simulink model "TST_Rail_CtlLoop"  (R2016b)
settings: Solver=FixedStepDiscrete  StartTime=0.0  StopTime=simTime  FixedStep=sampleTime  RelTol=1e-3
values from neighbouring files (symbols this model uses):
  testCase = 1    [initTST_Rail_CtlLoop_001.m]
libraries: simulink x6, UnitTest_Lib x4
settings Model: Creator=zhengjinyan  LastModifiedBy=zhengjinyan
settings DebuggingCC: SignalRangeChecking=error

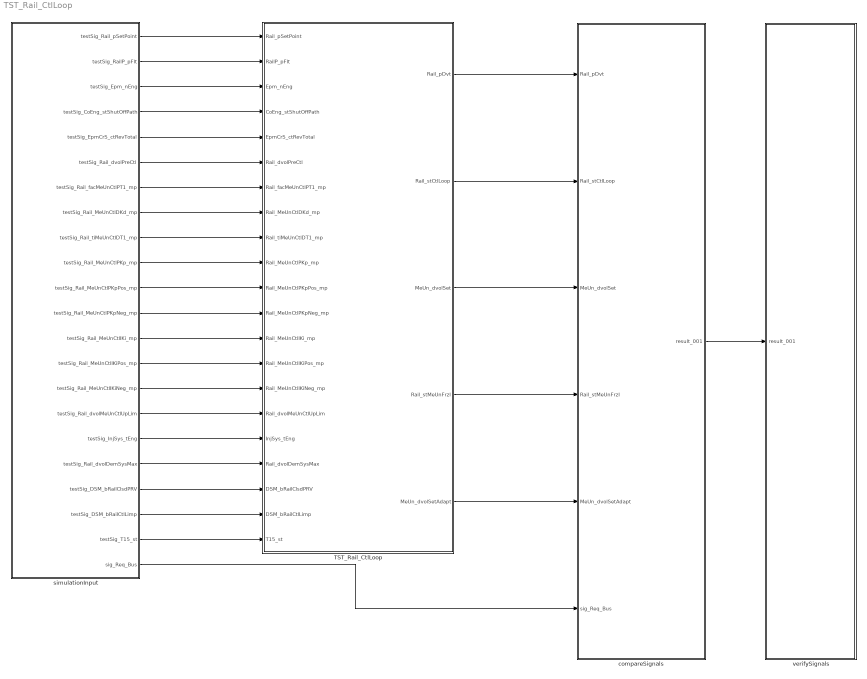
== system TST_Rail_CtlLoop ==
  TST_Rail_CtlLoop : Subsystem
  compareSignals : Subsystem
  simulationInput : Subsystem
  verifySignals : Subsystem
  wires:
  simulationInput/1(testSig_Rail_pSetPoint) -> TST_Rail_CtlLoop/1(Rail_pSetPoint)
  simulationInput/2(testSig_RailP_pFlt) -> TST_Rail_CtlLoop/2(RailP_pFlt)
  simulationInput/3(testSig_Epm_nEng) -> TST_Rail_CtlLoop/3(Epm_nEng)
  simulationInput/4(testSig_CoEng_stShutOffPath) -> TST_Rail_CtlLoop/4(CoEng_stShutOffPath)
  simulationInput/5(testSig_EpmCrS_ctRevTotal) -> TST_Rail_CtlLoop/5(EpmCrS_ctRevTotal)
  simulationInput/6(testSig_Rail_dvolPreCtl) -> TST_Rail_CtlLoop/6(Rail_dvolPreCtl)
  simulationInput/7(testSig_Rail_facMeUnCtlPT1_mp) -> TST_Rail_CtlLoop/7(Rail_facMeUnCtlPT1_mp)
  simulationInput/8(testSig_Rail_MeUnCtlDKd_mp) -> TST_Rail_CtlLoop/8(Rail_MeUnCtlDKd_mp)
  simulationInput/9(testSig_Rail_tiMeUnCtlDT1_mp) -> TST_Rail_CtlLoop/9(Rail_tiMeUnCtlDT1_mp)
  simulationInput/10(testSig_Rail_MeUnCtlPKp_mp) -> TST_Rail_CtlLoop/10(Rail_MeUnCtlPKp_mp)
  simulationInput/11(testSig_Rail_MeUnCtlPKpPos_mp) -> TST_Rail_CtlLoop/11(Rail_MeUnCtlPKpPos_mp)
  simulationInput/12(testSig_Rail_MeUnCtlPKpNeg_mp) -> TST_Rail_CtlLoop/12(Rail_MeUnCtlPKpNeg_mp)
  simulationInput/13(testSig_Rail_MeUnCtlIKi_mp) -> TST_Rail_CtlLoop/13(Rail_MeUnCtlIKi_mp)
  simulationInput/14(testSig_Rail_MeUnCtlIKiPos_mp) -> TST_Rail_CtlLoop/14(Rail_MeUnCtlIKiPos_mp)
  simulationInput/15(testSig_Rail_MeUnCtlIKiNeg_mp) -> TST_Rail_CtlLoop/15(Rail_MeUnCtlIKiNeg_mp)
  simulationInput/16(testSig_Rail_dvolMeUnCtlUpLim) -> TST_Rail_CtlLoop/16(Rail_dvolMeUnCtlUpLim)
  simulationInput/17(testSig_InjSys_tEng) -> TST_Rail_CtlLoop/17(InjSys_tEng)
  simulationInput/18(testSig_Rail_dvolDemSysMax) -> TST_Rail_CtlLoop/18(Rail_dvolDemSysMax)
  simulationInput/19(testSig_DSM_bRailClsdPRV) -> TST_Rail_CtlLoop/19(DSM_bRailClsdPRV)
  simulationInput/20(testSig_DSM_bRailCtlLimp) -> TST_Rail_CtlLoop/20(DSM_bRailCtlLimp)
  simulationInput/21(testSig_T15_st) -> TST_Rail_CtlLoop/21(T15_st)
  TST_Rail_CtlLoop/1(Rail_pDvt) -> compareSignals/1(Rail_pDvt)
  TST_Rail_CtlLoop/2(Rail_stCtlLoop) -> compareSignals/2(Rail_stCtlLoop)
  TST_Rail_CtlLoop/3(MeUn_dvolSet) -> compareSignals/3(MeUn_dvolSet)
  TST_Rail_CtlLoop/4(Rail_stMeUnFrzI) -> compareSignals/4(Rail_stMeUnFrzI)
  TST_Rail_CtlLoop/5(MeUn_dvolSetAdapt) -> compareSignals/5(MeUn_dvolSetAdapt)
  simulationInput/22(sig_Req_Bus) -> compareSignals/6(sig_Req_Bus)
  compareSignals/1(result_001) -> verifySignals/1(result_001)

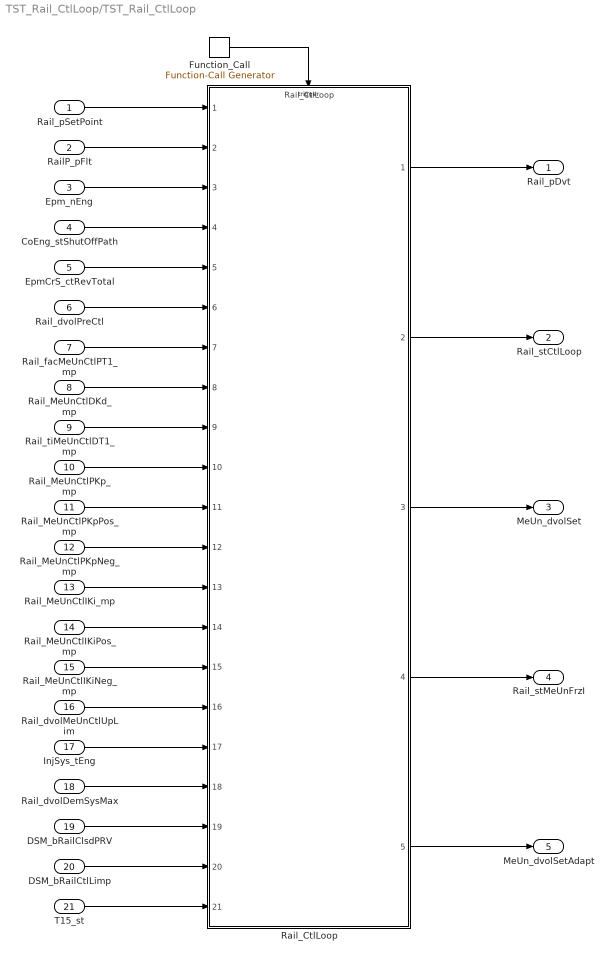
== system TST_Rail_CtlLoop/TST_Rail_CtlLoop ==
  Rail_pSetPoint : Inport
  RailP_pFlt : Inport  Port=2
  Epm_nEng : Inport  Port=3
  CoEng_stShutOffPath : Inport  Port=4
  EpmCrS_ctRevTotal : Inport  Port=5
  Rail_dvolPreCtl : Inport  Port=6
  Rail_facMeUnCtlPT1_mp : Inport  Port=7
  Rail_MeUnCtlDKd_mp : Inport  Port=8
  Rail_tiMeUnCtlDT1_mp : Inport  Port=9
  Rail_MeUnCtlPKp_mp : Inport  Port=10
  Rail_MeUnCtlPKpPos_mp : Inport  Port=11
  Rail_MeUnCtlPKpNeg_mp : Inport  Port=12
  Rail_MeUnCtlIKi_mp : Inport  Port=13
  Rail_MeUnCtlIKiPos_mp : Inport  Port=14
  Rail_MeUnCtlIKiNeg_mp : Inport  Port=15
  Rail_dvolMeUnCtlUpLim : Inport  Port=16
  InjSys_tEng : Inport  Port=17
  Rail_dvolDemSysMax : Inport  Port=18
  DSM_bRailClsdPRV : Inport  Port=19
  DSM_bRailCtlLimp : Inport  Port=20
  T15_st : Inport  Port=21
  Function_Call : simulink/Ports & Subsystems/Function-Call Generator  sample_time=sampleTime  numberOfIterations=1
  Rail_CtlLoop : ModelReference  ModelNameDialog=Rail_CtlLoop  SimulationMode=Normal  ModelReferenceVersion=1.34  TriggerPortName=function  TriggerPortTriggerType=function-call  TriggerPortStatesWhenEnabling=held
  Rail_pDvt : Outport
  Rail_stCtlLoop : Outport  Port=2
  MeUn_dvolSet : Outport  Port=3
  Rail_stMeUnFrzI : Outport  Port=4
  MeUn_dvolSetAdapt : Outport  Port=5
  wires:
  Function_Call/1 -> Rail_CtlLoop/Trigger
  Rail_pSetPoint/1 -> Rail_CtlLoop/1
  RailP_pFlt/1 -> Rail_CtlLoop/2
  Epm_nEng/1 -> Rail_CtlLoop/3
  CoEng_stShutOffPath/1 -> Rail_CtlLoop/4
  EpmCrS_ctRevTotal/1 -> Rail_CtlLoop/5
  Rail_dvolPreCtl/1 -> Rail_CtlLoop/6
  Rail_facMeUnCtlPT1_mp/1 -> Rail_CtlLoop/7
  Rail_MeUnCtlDKd_mp/1 -> Rail_CtlLoop/8
  Rail_tiMeUnCtlDT1_mp/1 -> Rail_CtlLoop/9
  Rail_MeUnCtlPKp_mp/1 -> Rail_CtlLoop/10
  Rail_MeUnCtlPKpPos_mp/1 -> Rail_CtlLoop/11
  Rail_MeUnCtlPKpNeg_mp/1 -> Rail_CtlLoop/12
  Rail_MeUnCtlIKi_mp/1 -> Rail_CtlLoop/13
  Rail_MeUnCtlIKiPos_mp/1 -> Rail_CtlLoop/14
  Rail_MeUnCtlIKiNeg_mp/1 -> Rail_CtlLoop/15
  Rail_dvolMeUnCtlUpLim/1 -> Rail_CtlLoop/16
  InjSys_tEng/1 -> Rail_CtlLoop/17
  Rail_dvolDemSysMax/1 -> Rail_CtlLoop/18
  DSM_bRailClsdPRV/1 -> Rail_CtlLoop/19
  DSM_bRailCtlLimp/1 -> Rail_CtlLoop/20
  T15_st/1 -> Rail_CtlLoop/21
  Rail_CtlLoop/1 -> Rail_pDvt/1
  Rail_CtlLoop/2 -> Rail_stCtlLoop/1
  Rail_CtlLoop/3 -> MeUn_dvolSet/1
  Rail_CtlLoop/4 -> Rail_stMeUnFrzI/1
  Rail_CtlLoop/5 -> MeUn_dvolSetAdapt/1

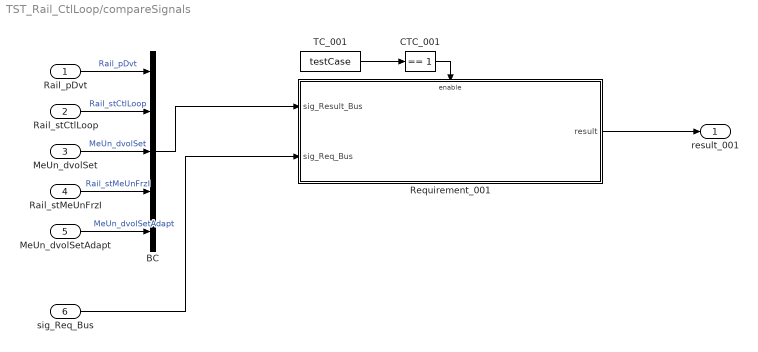
== system TST_Rail_CtlLoop/compareSignals ==
  Rail_pDvt : Inport
  Rail_stCtlLoop : Inport  Port=2
  MeUn_dvolSet : Inport  Port=3
  Rail_stMeUnFrzI : Inport  Port=4
  MeUn_dvolSetAdapt : Inport  Port=5
  sig_Req_Bus : Inport  Port=6
  BC : BusCreator  Inputs=5
  CTC_001 : simulink/Logic and Bit Operations/Compare To Constant  relop===  const=1  OutDataTypeStr=boolean
  Requirement_001 : Subsystem
  TC_001 : Constant  Value=testCase
  result_001 : Outport
  wires:
  Rail_pDvt/1 -> BC/1  "Rail_pDvt"
  Rail_stCtlLoop/1 -> BC/2  "Rail_stCtlLoop"
  MeUn_dvolSet/1 -> BC/3  "MeUn_dvolSet"
  Rail_stMeUnFrzI/1 -> BC/4  "Rail_stMeUnFrzI"
  MeUn_dvolSetAdapt/1 -> BC/5  "MeUn_dvolSetAdapt"
  TC_001/1 -> CTC_001/1
  CTC_001/1 -> Requirement_001/Enable
  sig_Req_Bus/1 -> Requirement_001/2(sig_Req_Bus)
  BC/1 -> Requirement_001/1(sig_Result_Bus)
  Requirement_001/1(result) -> result_001/1

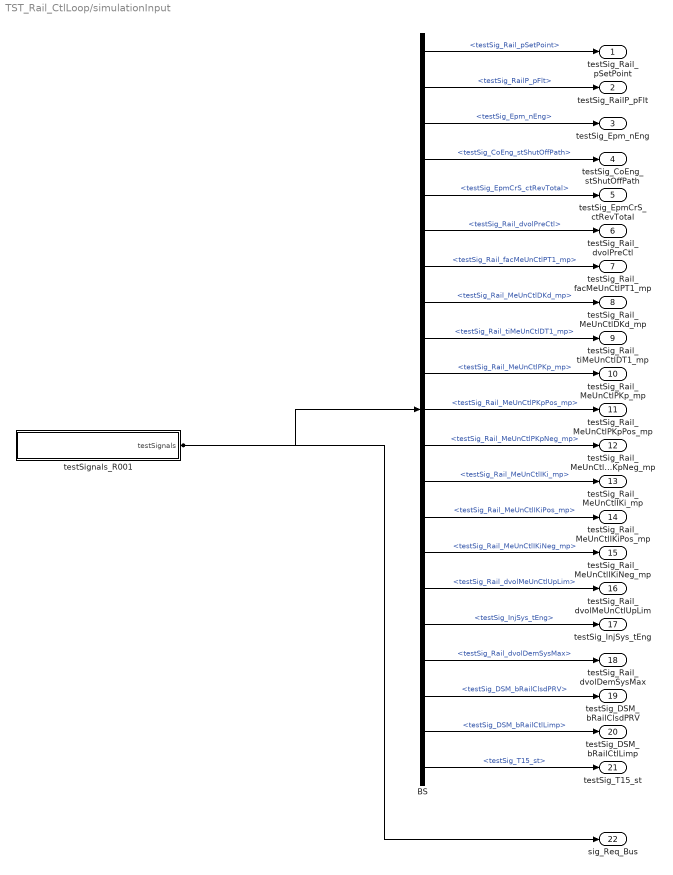
== system TST_Rail_CtlLoop/simulationInput ==
  BS : BusSelector  OutputSignals=testSig_Rail_pSetPoint,testSig_RailP_pFlt,testSig_Epm_nEng,testSig_CoEng_stShutOffPath,testSig_EpmCrS_ctRevTotal,testSig_Rail_dvolPreCtl,testSig_Rail_facMeUnCtlPT1_mp,testSig_Rail_MeUnCtlDKd_mp,testSig_Rail_tiMeUnCtlDT1_mp,testSig_Rail_MeUnCtlPKp_mp,testSig_Rail_MeUnCtlPKpPos_mp,testSig_Rail_MeUnCtlPKpNeg_mp,testSig_Rail_MeUnCtlIKi_mp,testSig_Rail_MeUnCtlIKiPos_mp,testSig_Rail_MeUnCtlIKiNeg_mp,testSig_Rail_dvolMeUnCtlUpLim,testSig_InjSys_tEng,testSig_Rail_dvolDemSysMax,testSig_DSM_bRailClsdPRV,testSig_DSM_bRailCtlLimp,testSig_T15_st
  testSignals_R001 : Subsystem
  testSig_Rail_pSetPoint : Outport
  testSig_RailP_pFlt : Outport  Port=2
  testSig_Epm_nEng : Outport  Port=3
  testSig_CoEng_stShutOffPath : Outport  Port=4
  testSig_EpmCrS_ctRevTotal : Outport  Port=5
  testSig_Rail_dvolPreCtl : Outport  Port=6
  testSig_Rail_facMeUnCtlPT1_mp : Outport  Port=7
  testSig_Rail_MeUnCtlDKd_mp : Outport  Port=8
  testSig_Rail_tiMeUnCtlDT1_mp : Outport  Port=9
  testSig_Rail_MeUnCtlPKp_mp : Outport  Port=10
  testSig_Rail_MeUnCtlPKpPos_mp : Outport  Port=11
  testSig_Rail_MeUnCtlPKpNeg_mp : Outport  Port=12
  testSig_Rail_MeUnCtlIKi_mp : Outport  Port=13
  testSig_Rail_MeUnCtlIKiPos_mp : Outport  Port=14
  testSig_Rail_MeUnCtlIKiNeg_mp : Outport  Port=15
  testSig_Rail_dvolMeUnCtlUpLim : Outport  Port=16
  testSig_InjSys_tEng : Outport  Port=17
  testSig_Rail_dvolDemSysMax : Outport  Port=18
  testSig_DSM_bRailClsdPRV : Outport  Port=19
  testSig_DSM_bRailCtlLimp : Outport  Port=20
  testSig_T15_st : Outport  Port=21
  sig_Req_Bus : Outport  Port=22
  wires:
  BS/1 -> testSig_Rail_pSetPoint/1  "<testSig_Rail_pSetPoint>"
  BS/2 -> testSig_RailP_pFlt/1  "<testSig_RailP_pFlt>"
  BS/3 -> testSig_Epm_nEng/1  "<testSig_Epm_nEng>"
  BS/4 -> testSig_CoEng_stShutOffPath/1  "<testSig_CoEng_stShutOffPath>"
  BS/5 -> testSig_EpmCrS_ctRevTotal/1  "<testSig_EpmCrS_ctRevTotal>"
  BS/6 -> testSig_Rail_dvolPreCtl/1  "<testSig_Rail_dvolPreCtl>"
  BS/7 -> testSig_Rail_facMeUnCtlPT1_mp/1  "<testSig_Rail_facMeUnCtlPT1_mp>"
  BS/8 -> testSig_Rail_MeUnCtlDKd_mp/1  "<testSig_Rail_MeUnCtlDKd_mp>"
  BS/9 -> testSig_Rail_tiMeUnCtlDT1_mp/1  "<testSig_Rail_tiMeUnCtlDT1_mp>"
  BS/10 -> testSig_Rail_MeUnCtlPKp_mp/1  "<testSig_Rail_MeUnCtlPKp_mp>"
  BS/11 -> testSig_Rail_MeUnCtlPKpPos_mp/1  "<testSig_Rail_MeUnCtlPKpPos_mp>"
  BS/12 -> testSig_Rail_MeUnCtlPKpNeg_mp/1  "<testSig_Rail_MeUnCtlPKpNeg_mp>"
  BS/13 -> testSig_Rail_MeUnCtlIKi_mp/1  "<testSig_Rail_MeUnCtlIKi_mp>"
  BS/14 -> testSig_Rail_MeUnCtlIKiPos_mp/1  "<testSig_Rail_MeUnCtlIKiPos_mp>"
  BS/15 -> testSig_Rail_MeUnCtlIKiNeg_mp/1  "<testSig_Rail_MeUnCtlIKiNeg_mp>"
  BS/16 -> testSig_Rail_dvolMeUnCtlUpLim/1  "<testSig_Rail_dvolMeUnCtlUpLim>"
  BS/17 -> testSig_InjSys_tEng/1  "<testSig_InjSys_tEng>"
  BS/18 -> testSig_Rail_dvolDemSysMax/1  "<testSig_Rail_dvolDemSysMax>"
  BS/19 -> testSig_DSM_bRailClsdPRV/1  "<testSig_DSM_bRailClsdPRV>"
  BS/20 -> testSig_DSM_bRailCtlLimp/1  "<testSig_DSM_bRailCtlLimp>"
  BS/21 -> testSig_T15_st/1  "<testSig_T15_st>"
  testSignals_R001/1(testSignals) -> BS/1, sig_Req_Bus/1

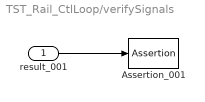
== system TST_Rail_CtlLoop/verifySignals ==
  result_001 : Inport
  Assertion_001 : Assertion  Enabled=off
  wires:
  result_001/1 -> Assertion_001/1

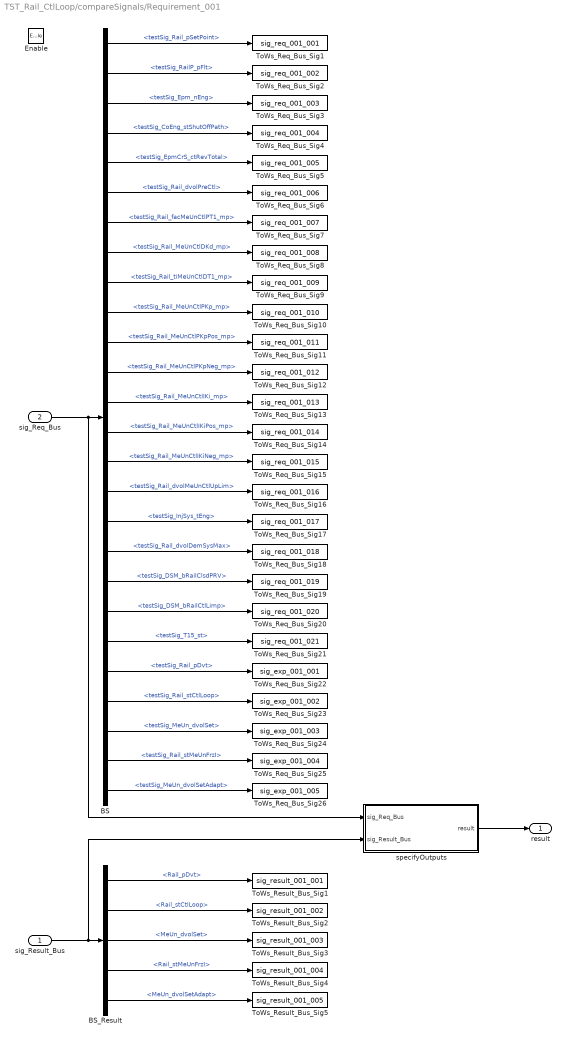
== system TST_Rail_CtlLoop/compareSignals/Requirement_001 ==
  sig_Result_Bus : Inport
  sig_Req_Bus : Inport  Port=2
  Enable : EnablePort
  BS : BusSelector  OutputSignals=testSig_Rail_pSetPoint,testSig_RailP_pFlt,testSig_Epm_nEng,testSig_CoEng_stShutOffPath,testSig_EpmCrS_ctRevTotal,testSig_Rail_dvolPreCtl,testSig_Rail_facMeUnCtlPT1_mp,testSig_Rail_MeUnCtlDKd_mp,testSig_Rail_tiMeUnCtlDT1_mp,testSig_Rail_MeUnCtlPKp_mp,testSig_Rail_MeUnCtlPKpPos_mp,testSig_Rail_MeUnCtlPKpNeg_mp,testSig_Rail_MeUnCtlIKi_mp,testSig_Rail_MeUnCtlIKiPos_mp,testSig_Rail_MeUnCtlIKiNeg_mp,testSig_Rail_dvolMeUnCtlUpLim,testSig_InjSys_tEng,testSig_Rail_dvolDemSysMax,testSig_DSM_bRailClsdPRV,testSig_DSM_bRailCtlLimp,testSig_T15_st,testSig_Rail_pDvt,testSig_Rail_stCtlLoop,testSig_MeUn_dvolSet,testSig_Rail_stMeUnFrzI,testSig_MeUn_dvolSetAdapt
  BS_Result : BusSelector  OutputSignals=Rail_pDvt,Rail_stCtlLoop,MeUn_dvolSet,Rail_stMeUnFrzI,MeUn_dvolSetAdapt
  ToWs_Req_Bus_Sig1 : ToWorkspace  VariableName=sig_req_001_001  SaveFormat=Structure With Time
  ToWs_Req_Bus_Sig10 : ToWorkspace  VariableName=sig_req_001_010  SaveFormat=Structure With Time
  ToWs_Req_Bus_Sig11 : ToWorkspace  VariableName=sig_req_001_011  SaveFormat=Structure With Time
  ToWs_Req_Bus_Sig12 : ToWorkspace  VariableName=sig_req_001_012  SaveFormat=Structure With Time
  ToWs_Req_Bus_Sig13 : ToWorkspace  VariableName=sig_req_001_013  SaveFormat=Structure With Time
  ToWs_Req_Bus_Sig14 : ToWorkspace  VariableName=sig_req_001_014  SaveFormat=Structure With Time
  ToWs_Req_Bus_Sig15 : ToWorkspace  VariableName=sig_req_001_015  SaveFormat=Structure With Time
  ToWs_Req_Bus_Sig16 : ToWorkspace  VariableName=sig_req_001_016  SaveFormat=Structure With Time
  ToWs_Req_Bus_Sig17 : ToWorkspace  VariableName=sig_req_001_017  SaveFormat=Structure With Time
  ToWs_Req_Bus_Sig18 : ToWorkspace  VariableName=sig_req_001_018  SaveFormat=Structure With Time
  ToWs_Req_Bus_Sig19 : ToWorkspace  VariableName=sig_req_001_019  SaveFormat=Structure With Time
  ToWs_Req_Bus_Sig2 : ToWorkspace  VariableName=sig_req_001_002  SaveFormat=Structure With Time
  ToWs_Req_Bus_Sig20 : ToWorkspace  VariableName=sig_req_001_020  SaveFormat=Structure With Time
  ToWs_Req_Bus_Sig21 : ToWorkspace  VariableName=sig_req_001_021  SaveFormat=Structure With Time
  ToWs_Req_Bus_Sig22 : ToWorkspace  VariableName=sig_exp_001_001  SaveFormat=Structure With Time
  ToWs_Req_Bus_Sig23 : ToWorkspace  VariableName=sig_exp_001_002  SaveFormat=Structure With Time
  ToWs_Req_Bus_Sig24 : ToWorkspace  VariableName=sig_exp_001_003  SaveFormat=Structure With Time
  ToWs_Req_Bus_Sig25 : ToWorkspace  VariableName=sig_exp_001_004  SaveFormat=Structure With Time
  ToWs_Req_Bus_Sig26 : ToWorkspace  VariableName=sig_exp_001_005  SaveFormat=Structure With Time
  ToWs_Req_Bus_Sig3 : ToWorkspace  VariableName=sig_req_001_003  SaveFormat=Structure With Time
  ToWs_Req_Bus_Sig4 : ToWorkspace  VariableName=sig_req_001_004  SaveFormat=Structure With Time
  ToWs_Req_Bus_Sig5 : ToWorkspace  VariableName=sig_req_001_005  SaveFormat=Structure With Time
  ToWs_Req_Bus_Sig6 : ToWorkspace  VariableName=sig_req_001_006  SaveFormat=Structure With Time
  ToWs_Req_Bus_Sig7 : ToWorkspace  VariableName=sig_req_001_007  SaveFormat=Structure With Time
  ToWs_Req_Bus_Sig8 : ToWorkspace  VariableName=sig_req_001_008  SaveFormat=Structure With Time
  ToWs_Req_Bus_Sig9 : ToWorkspace  VariableName=sig_req_001_009  SaveFormat=Structure With Time
  ToWs_Result_Bus_Sig1 : ToWorkspace  VariableName=sig_result_001_001  SaveFormat=Structure With Time
  ToWs_Result_Bus_Sig2 : ToWorkspace  VariableName=sig_result_001_002  SaveFormat=Structure With Time
  ToWs_Result_Bus_Sig3 : ToWorkspace  VariableName=sig_result_001_003  SaveFormat=Structure With Time
  ToWs_Result_Bus_Sig4 : ToWorkspace  VariableName=sig_result_001_004  SaveFormat=Structure With Time
  ToWs_Result_Bus_Sig5 : ToWorkspace  VariableName=sig_result_001_005  SaveFormat=Structure With Time
  specifyOutputs : Subsystem
  result : Outport
  wires:
  sig_Req_Bus/1 -> BS/1, specifyOutputs/1(sig_Req_Bus)
  BS/1 -> ToWs_Req_Bus_Sig1/1  "<testSig_Rail_pSetPoint>"
  BS/2 -> ToWs_Req_Bus_Sig2/1  "<testSig_RailP_pFlt>"
  BS/3 -> ToWs_Req_Bus_Sig3/1  "<testSig_Epm_nEng>"
  BS/4 -> ToWs_Req_Bus_Sig4/1  "<testSig_CoEng_stShutOffPath>"
  BS/5 -> ToWs_Req_Bus_Sig5/1  "<testSig_EpmCrS_ctRevTotal>"
  BS/6 -> ToWs_Req_Bus_Sig6/1  "<testSig_Rail_dvolPreCtl>"
  BS/7 -> ToWs_Req_Bus_Sig7/1  "<testSig_Rail_facMeUnCtlPT1_mp>"
  BS/8 -> ToWs_Req_Bus_Sig8/1  "<testSig_Rail_MeUnCtlDKd_mp>"
  BS/9 -> ToWs_Req_Bus_Sig9/1  "<testSig_Rail_tiMeUnCtlDT1_mp>"
  BS/10 -> ToWs_Req_Bus_Sig10/1  "<testSig_Rail_MeUnCtlPKp_mp>"
  BS/11 -> ToWs_Req_Bus_Sig11/1  "<testSig_Rail_MeUnCtlPKpPos_mp>"
  BS/12 -> ToWs_Req_Bus_Sig12/1  "<testSig_Rail_MeUnCtlPKpNeg_mp>"
  BS/13 -> ToWs_Req_Bus_Sig13/1  "<testSig_Rail_MeUnCtlIKi_mp>"
  BS/14 -> ToWs_Req_Bus_Sig14/1  "<testSig_Rail_MeUnCtlIKiPos_mp>"
  BS/15 -> ToWs_Req_Bus_Sig15/1  "<testSig_Rail_MeUnCtlIKiNeg_mp>"
  BS/16 -> ToWs_Req_Bus_Sig16/1  "<testSig_Rail_dvolMeUnCtlUpLim>"
  BS/17 -> ToWs_Req_Bus_Sig17/1  "<testSig_InjSys_tEng>"
  BS/18 -> ToWs_Req_Bus_Sig18/1  "<testSig_Rail_dvolDemSysMax>"
  BS/19 -> ToWs_Req_Bus_Sig19/1  "<testSig_DSM_bRailClsdPRV>"
  BS/20 -> ToWs_Req_Bus_Sig20/1  "<testSig_DSM_bRailCtlLimp>"
  BS/21 -> ToWs_Req_Bus_Sig21/1  "<testSig_T15_st>"
  BS/22 -> ToWs_Req_Bus_Sig22/1  "<testSig_Rail_pDvt>"
  BS/23 -> ToWs_Req_Bus_Sig23/1  "<testSig_Rail_stCtlLoop>"
  BS/24 -> ToWs_Req_Bus_Sig24/1  "<testSig_MeUn_dvolSet>"
  BS/25 -> ToWs_Req_Bus_Sig25/1  "<testSig_Rail_stMeUnFrzI>"
  BS/26 -> ToWs_Req_Bus_Sig26/1  "<testSig_MeUn_dvolSetAdapt>"
  sig_Result_Bus/1 -> BS_Result/1, specifyOutputs/2(sig_Result_Bus)
  BS_Result/1 -> ToWs_Result_Bus_Sig1/1  "<Rail_pDvt>"
  BS_Result/2 -> ToWs_Result_Bus_Sig2/1  "<Rail_stCtlLoop>"
  BS_Result/3 -> ToWs_Result_Bus_Sig3/1  "<MeUn_dvolSet>"
  BS_Result/4 -> ToWs_Result_Bus_Sig4/1  "<Rail_stMeUnFrzI>"
  BS_Result/5 -> ToWs_Result_Bus_Sig5/1  "<MeUn_dvolSetAdapt>"
  specifyOutputs/1(result) -> result/1

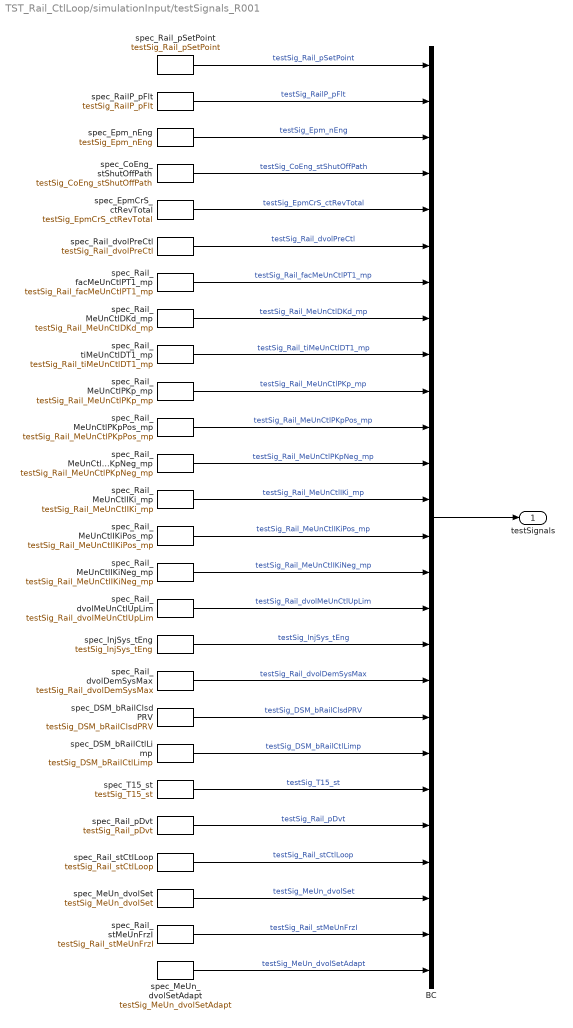
== system TST_Rail_CtlLoop/simulationInput/testSignals_R001 ==
  BC : BusCreator  Inputs=26
  spec_CoEng_stShutOffPath : FromWorkspace  VariableName=testSig_CoEng_stShutOffPath  Interpolate=off  OutputAfterFinalValue=Holding final value
  spec_DSM_bRailClsdPRV : FromWorkspace  VariableName=testSig_DSM_bRailClsdPRV  Interpolate=off  OutputAfterFinalValue=Holding final value
  spec_DSM_bRailCtlLimp : FromWorkspace  VariableName=testSig_DSM_bRailCtlLimp  Interpolate=off  OutputAfterFinalValue=Holding final value
  spec_EpmCrS_ctRevTotal : FromWorkspace  VariableName=testSig_EpmCrS_ctRevTotal  Interpolate=off  OutputAfterFinalValue=Holding final value
  spec_Epm_nEng : FromWorkspace  VariableName=testSig_Epm_nEng  Interpolate=off  OutputAfterFinalValue=Holding final value
  spec_InjSys_tEng : FromWorkspace  VariableName=testSig_InjSys_tEng  Interpolate=off  OutputAfterFinalValue=Holding final value
  spec_MeUn_dvolSet : FromWorkspace  VariableName=testSig_MeUn_dvolSet  Interpolate=off  OutputAfterFinalValue=Holding final value
  spec_MeUn_dvolSetAdapt : FromWorkspace  VariableName=testSig_MeUn_dvolSetAdapt  Interpolate=off  OutputAfterFinalValue=Holding final value
  spec_RailP_pFlt : FromWorkspace  VariableName=testSig_RailP_pFlt  Interpolate=off  OutputAfterFinalValue=Holding final value
  spec_Rail_MeUnCtlDKd_mp : FromWorkspace  VariableName=testSig_Rail_MeUnCtlDKd_mp  Interpolate=off  OutputAfterFinalValue=Holding final value
  spec_Rail_MeUnCtlIKiNeg_mp : FromWorkspace  VariableName=testSig_Rail_MeUnCtlIKiNeg_mp  Interpolate=off  OutputAfterFinalValue=Holding final value
  spec_Rail_MeUnCtlIKiPos_mp : FromWorkspace  VariableName=testSig_Rail_MeUnCtlIKiPos_mp  Interpolate=off  OutputAfterFinalValue=Holding final value
  spec_Rail_MeUnCtlIKi_mp : FromWorkspace  VariableName=testSig_Rail_MeUnCtlIKi_mp  Interpolate=off  OutputAfterFinalValue=Holding final value
  spec_Rail_MeUnCtlPKpNeg_mp : FromWorkspace  VariableName=testSig_Rail_MeUnCtlPKpNeg_mp  Interpolate=off  OutputAfterFinalValue=Holding final value
  spec_Rail_MeUnCtlPKpPos_mp : FromWorkspace  VariableName=testSig_Rail_MeUnCtlPKpPos_mp  Interpolate=off  OutputAfterFinalValue=Holding final value
  spec_Rail_MeUnCtlPKp_mp : FromWorkspace  VariableName=testSig_Rail_MeUnCtlPKp_mp  Interpolate=off  OutputAfterFinalValue=Holding final value
  spec_Rail_dvolDemSysMax : FromWorkspace  VariableName=testSig_Rail_dvolDemSysMax  Interpolate=off  OutputAfterFinalValue=Holding final value
  spec_Rail_dvolMeUnCtlUpLim : FromWorkspace  VariableName=testSig_Rail_dvolMeUnCtlUpLim  Interpolate=off  OutputAfterFinalValue=Holding final value
  spec_Rail_dvolPreCtl : FromWorkspace  VariableName=testSig_Rail_dvolPreCtl  Interpolate=off  OutputAfterFinalValue=Holding final value
  spec_Rail_facMeUnCtlPT1_mp : FromWorkspace  VariableName=testSig_Rail_facMeUnCtlPT1_mp  Interpolate=off  OutputAfterFinalValue=Holding final value
  spec_Rail_pDvt : FromWorkspace  VariableName=testSig_Rail_pDvt  Interpolate=off  OutputAfterFinalValue=Holding final value
  spec_Rail_pSetPoint : FromWorkspace  VariableName=testSig_Rail_pSetPoint  Interpolate=off  OutputAfterFinalValue=Holding final value
  spec_Rail_stCtlLoop : FromWorkspace  VariableName=testSig_Rail_stCtlLoop  Interpolate=off  OutputAfterFinalValue=Holding final value
  spec_Rail_stMeUnFrzI : FromWorkspace  VariableName=testSig_Rail_stMeUnFrzI  Interpolate=off  OutputAfterFinalValue=Holding final value
  spec_Rail_tiMeUnCtlDT1_mp : FromWorkspace  VariableName=testSig_Rail_tiMeUnCtlDT1_mp  Interpolate=off  OutputAfterFinalValue=Holding final value
  spec_T15_st : FromWorkspace  VariableName=testSig_T15_st  Interpolate=off  OutputAfterFinalValue=Holding final value
  testSignals : Outport
  wires:
  BC/1 -> testSignals/1
  spec_Rail_pSetPoint/1 -> BC/1  "testSig_Rail_pSetPoint"
  spec_RailP_pFlt/1 -> BC/2  "testSig_RailP_pFlt"
  spec_Epm_nEng/1 -> BC/3  "testSig_Epm_nEng"
  spec_CoEng_stShutOffPath/1 -> BC/4  "testSig_CoEng_stShutOffPath"
  spec_EpmCrS_ctRevTotal/1 -> BC/5  "testSig_EpmCrS_ctRevTotal"
  spec_Rail_dvolPreCtl/1 -> BC/6  "testSig_Rail_dvolPreCtl"
  spec_Rail_facMeUnCtlPT1_mp/1 -> BC/7  "testSig_Rail_facMeUnCtlPT1_mp"
  spec_Rail_MeUnCtlDKd_mp/1 -> BC/8  "testSig_Rail_MeUnCtlDKd_mp"
  spec_Rail_tiMeUnCtlDT1_mp/1 -> BC/9  "testSig_Rail_tiMeUnCtlDT1_mp"
  spec_Rail_MeUnCtlPKp_mp/1 -> BC/10  "testSig_Rail_MeUnCtlPKp_mp"
  spec_Rail_MeUnCtlPKpPos_mp/1 -> BC/11  "testSig_Rail_MeUnCtlPKpPos_mp"
  spec_Rail_MeUnCtlPKpNeg_mp/1 -> BC/12  "testSig_Rail_MeUnCtlPKpNeg_mp"
  spec_Rail_MeUnCtlIKi_mp/1 -> BC/13  "testSig_Rail_MeUnCtlIKi_mp"
  spec_Rail_MeUnCtlIKiPos_mp/1 -> BC/14  "testSig_Rail_MeUnCtlIKiPos_mp"
  spec_Rail_MeUnCtlIKiNeg_mp/1 -> BC/15  "testSig_Rail_MeUnCtlIKiNeg_mp"
  spec_Rail_dvolMeUnCtlUpLim/1 -> BC/16  "testSig_Rail_dvolMeUnCtlUpLim"
  spec_InjSys_tEng/1 -> BC/17  "testSig_InjSys_tEng"
  spec_Rail_dvolDemSysMax/1 -> BC/18  "testSig_Rail_dvolDemSysMax"
  spec_DSM_bRailClsdPRV/1 -> BC/19  "testSig_DSM_bRailClsdPRV"
  spec_DSM_bRailCtlLimp/1 -> BC/20  "testSig_DSM_bRailCtlLimp"
  spec_T15_st/1 -> BC/21  "testSig_T15_st"
  spec_Rail_pDvt/1 -> BC/22  "testSig_Rail_pDvt"
  spec_Rail_stCtlLoop/1 -> BC/23  "testSig_Rail_stCtlLoop"
  spec_MeUn_dvolSet/1 -> BC/24  "testSig_MeUn_dvolSet"
  spec_Rail_stMeUnFrzI/1 -> BC/25  "testSig_Rail_stMeUnFrzI"
  spec_MeUn_dvolSetAdapt/1 -> BC/26  "testSig_MeUn_dvolSetAdapt"

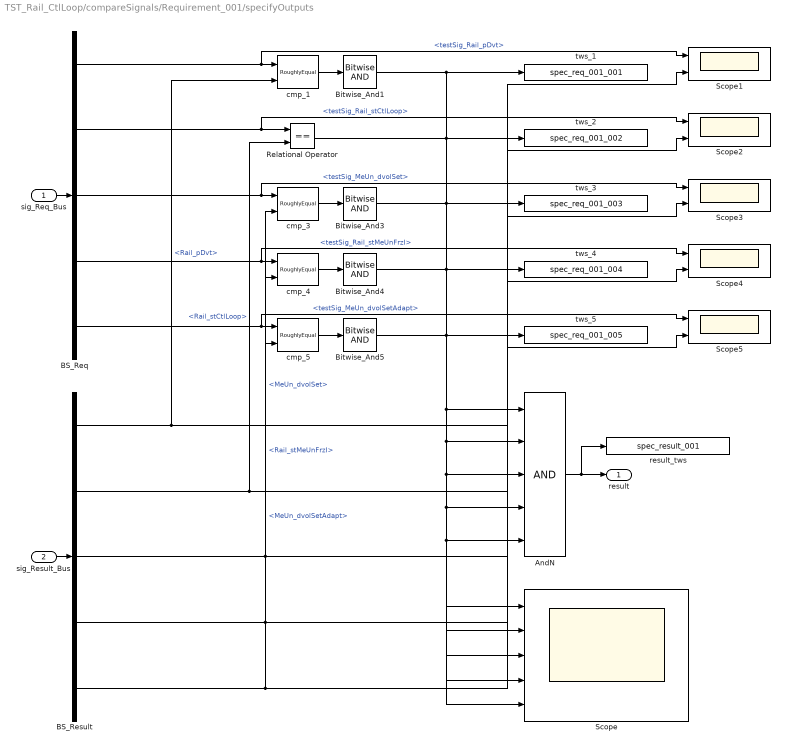
== system TST_Rail_CtlLoop/compareSignals/Requirement_001/specifyOutputs ==
  sig_Req_Bus : Inport
  sig_Result_Bus : Inport  Port=2
  AndN : Logic  Inputs=5
  BS_Req : BusSelector  OutputSignals=testSig_Rail_pDvt,testSig_Rail_stCtlLoop,testSig_MeUn_dvolSet,testSig_Rail_stMeUnFrzI,testSig_MeUn_dvolSetAdapt
  BS_Result : BusSelector  OutputSignals=Rail_pDvt,Rail_stCtlLoop,MeUn_dvolSet,Rail_stMeUnFrzI,MeUn_dvolSetAdapt
  Bitwise_And{1,3..5} (4 alike) : simulink/Logic and Bit Operations/Bitwise Operator  logicop=AND  UseBitMask=off  BitMask=bin2dec('11011001')  BitMaskRealWorld=Stored Integer
  Relational Operator : RelationalOperator  Operator===  OutDataTypeStr=boolean  RndMeth=Simplest
  Scope : Scope  NumInputPorts=5
  Scope{1..5} (5 alike) : Scope  NumInputPorts=2
  cmp_{1,3..5} (4 alike) : UnitTest_Lib/RoughlyEqual  slope=0.1
  result_tws : ToWorkspace  VariableName=spec_result_001
  tws_1 : ToWorkspace  VariableName=spec_req_001_001
  tws_2 : ToWorkspace  VariableName=spec_req_001_002
  tws_3 : ToWorkspace  VariableName=spec_req_001_003
  tws_4 : ToWorkspace  VariableName=spec_req_001_004
  tws_5 : ToWorkspace  VariableName=spec_req_001_005
  result : Outport
  wires:
  sig_Req_Bus/1 -> BS_Req/1
  sig_Result_Bus/1 -> BS_Result/1
  AndN/1 -> result/1, result_tws/1
  BS_Req/1 -> cmp_1/1, Scope1/1  "<testSig_Rail_pDvt>"
  BS_Result/1 -> cmp_1/2, Scope1/2  "<Rail_pDvt>"
  cmp_1/1 -> Bitwise_And1/1
  Bitwise_And1/1 -> AndN/1, Scope/1, tws_1/1
  BS_Req/2 -> Relational Operator/1, Scope2/1  "<testSig_Rail_stCtlLoop>"
  BS_Result/2 -> Scope2/2, Relational Operator/2  "<Rail_stCtlLoop>"
  Relational Operator/1 -> AndN/2, Scope/2, tws_2/1
  BS_Req/3 -> cmp_3/1, Scope3/1  "<testSig_MeUn_dvolSet>"
  BS_Result/3 -> cmp_3/2, Scope3/2  "<MeUn_dvolSet>"
  cmp_3/1 -> Bitwise_And3/1
  Bitwise_And3/1 -> AndN/3, Scope/3, tws_3/1
  BS_Req/4 -> cmp_4/1, Scope4/1  "<testSig_Rail_stMeUnFrzI>"
  BS_Result/4 -> cmp_4/2, Scope4/2  "<Rail_stMeUnFrzI>"
  cmp_4/1 -> Bitwise_And4/1
  Bitwise_And4/1 -> AndN/4, Scope/4, tws_4/1
  BS_Req/5 -> cmp_5/1, Scope5/1  "<testSig_MeUn_dvolSetAdapt>"
  BS_Result/5 -> cmp_5/2, Scope5/2  "<MeUn_dvolSetAdapt>"
  cmp_5/1 -> Bitwise_And5/1
  Bitwise_And5/1 -> AndN/5, Scope/5, tws_5/1
